simulink model "fan_control_Old"  (R2024b)
settings: Solver=VariableStepAuto  StartTime=0.0  StopTime=inf  FixedStep=1e-4  MaxStep=1e-4  RelTol=1e-6
values from neighbouring files (symbols this model uses):
  a = 0.0    [data.sldd]
  J_f = 0.0    [data.sldd]
  J_m = 0.0    [data.sldd]
  PID_I = 0.03    [data.sldd]
  PID_P = 0.06    [data.sldd]
  RateSpeed = 0.0    [data.sldd]
  RateTorque = 0.0    [data.sldd]
  Reference_Speed = 0.0    [data.sldd]
  Speed_max = 0.0    [data.sldd]
  T0 = 0.0    [data.sldd]
  Torque_max = 0.0    [data.sldd]
settings Model: DataDictionary=data.sldd  Creator=SESA504213  LastModifiedBy=SESA504213

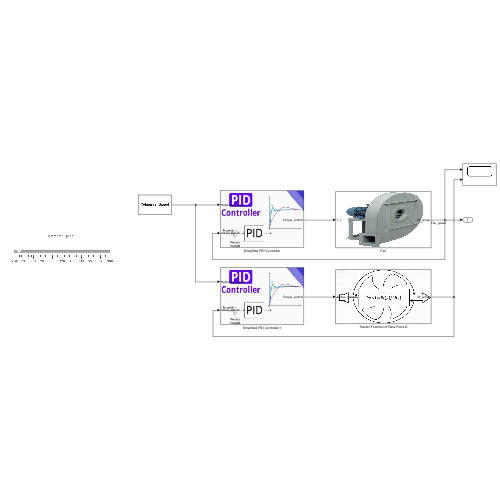
[thumbnail: Simulink's stored preview of the top-level diagram]
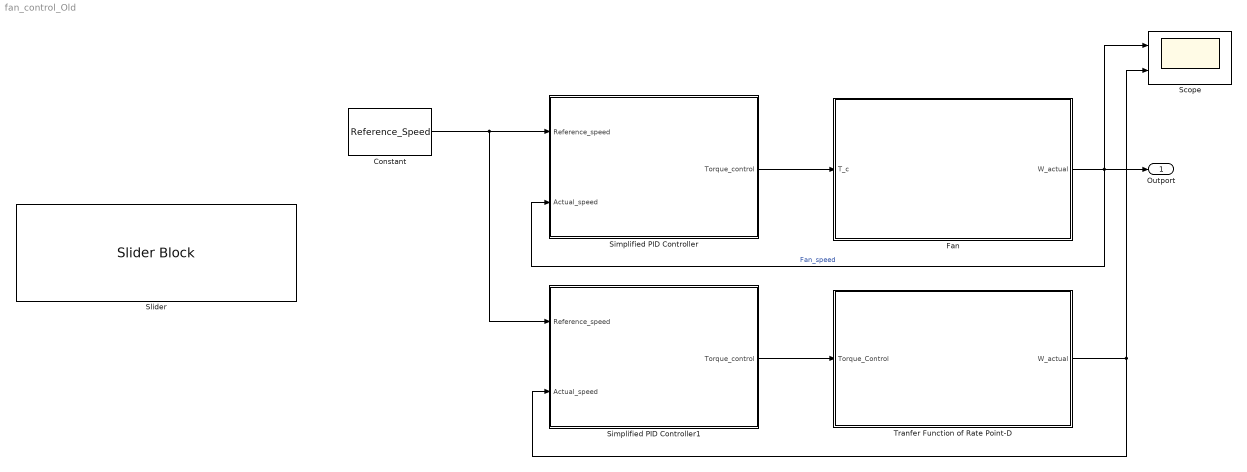
== system fan_control_Old ==
  Constant : Constant  Value=Reference_Speed
  Fan : Subsystem
      mask Display: image('FanwithMotor.jpg');
  Scope : Scope  NumInputPorts=2
  Simplified PID Controller : Subsystem
      mask Display: image('PIDController.jpg');
  Simplified PID Controller1 : Subsystem
      mask Display: image('PIDController.jpg');
  Slider : SliderBlock  ScaleMin=250  ScaleMax=390
  Tranfer Function of Rate Point-D : Subsystem
      mask Display: image('TransferFcn.jpg');
  Outport : Outport
  wires:
  Fan/1(W_actual) -> Outport/1, Simplified PID Controller/2(Actual_speed), Scope/1  "Fan_speed"
  Simplified PID Controller/1(Torque_control) -> Fan/1(T_c)
  Constant/1 -> Simplified PID Controller1/1(Reference_speed), Simplified PID Controller/1(Reference_speed)
  Simplified PID Controller1/1(Torque_control) -> Tranfer Function of Rate Point-D/1(Torque_Control)
  Tranfer Function of Rate Point-D/1(W_actual) -> Simplified PID Controller1/2(Actual_speed), Scope/2

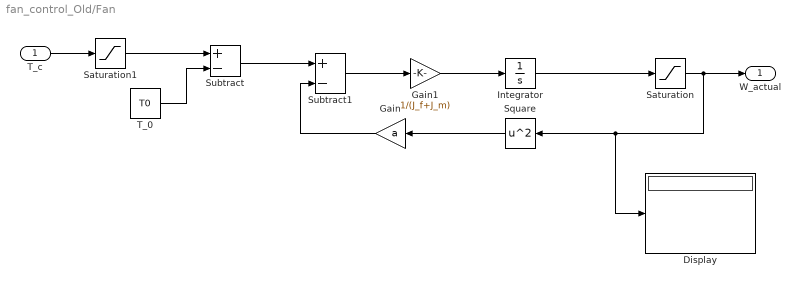
== system fan_control_Old/Fan ==
  T_c : Inport
  Display : Display
  Gain : Gain  Gain=a
  Gain1 : Gain  Gain=1/(J_f+J_m)
  Integrator : Integrator
  Saturation : Saturate  UpperLimit=Speed_max  LowerLimit=-Speed_max
  Saturation1 : Saturate  UpperLimit=Torque_max  LowerLimit=-Torque_max
  Square : Math  Operator=square
  Subtract : Sum  Inputs=+-
  Subtract1 : Sum  Inputs=+-
  T_0 : Constant  Value=T0
  W_actual : Outport
  wires:
  Gain1/1 -> Integrator/1
  Square/1 -> Gain/1
  T_c/1 -> Saturation1/1
  T_0/1 -> Subtract/2
  Subtract1/1 -> Gain1/1
  Integrator/1 -> Saturation/1
  Subtract/1 -> Subtract1/1
  Gain/1 -> Subtract1/2
  Saturation/1 -> Display/1, Square/1, W_actual/1
  Saturation1/1 -> Subtract/1

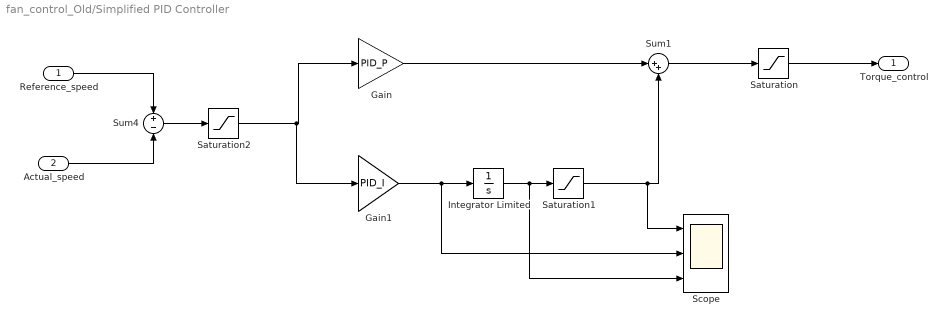
== system fan_control_Old/Simplified PID Controller ==
  Reference_speed : Inport
  Actual_speed : Inport  Port=2
  Gain : Gain  Gain=PID_P
  Gain1 : Gain  Gain=PID_I
  Integrator Limited : Integrator  LimitOutput=on  UpperSaturationLimit=RateTorque  LowerSaturationLimit=-RateTorque
  Saturation : Saturate  UpperLimit=Torque_max  LowerLimit=-Torque_max
  Saturation1 : Saturate  UpperLimit=Torque_max  LowerLimit=-Torque_max
  Saturation2 : Saturate  UpperLimit=Speed_max  LowerLimit=-Speed_max
  Scope : Scope  NumInputPorts=3
  Sum1 : Sum  Inputs=|++
  Sum4 : Sum  Inputs=+-
  Torque_control : Outport
  wires:
  Gain1/1 -> Integrator Limited/1, Scope/2
  Gain/1 -> Sum1/1
  Sum1/1 -> Saturation/1
  Integrator Limited/1 -> Scope/3, Saturation1/1
  Saturation1/1 -> Scope/1, Sum1/2
  Saturation/1 -> Torque_control/1
  Reference_speed/1 -> Sum4/1
  Actual_speed/1 -> Sum4/2
  Saturation2/1 -> Gain1/1, Gain/1
  Sum4/1 -> Saturation2/1

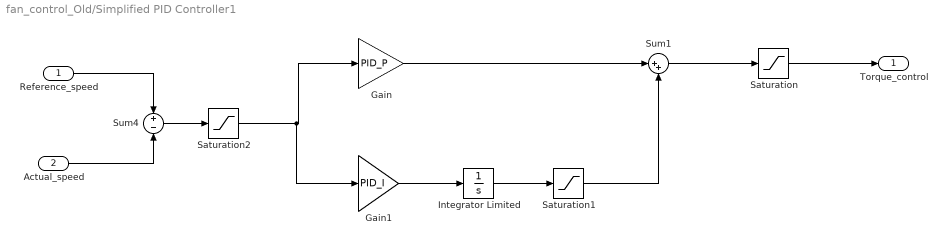
== system fan_control_Old/Simplified PID Controller1 ==
  Reference_speed : Inport
  Actual_speed : Inport  Port=2
  Gain : Gain  Gain=PID_P
  Gain1 : Gain  Gain=PID_I
  Integrator Limited : Integrator  LimitOutput=on  UpperSaturationLimit=RateTorque  LowerSaturationLimit=-RateTorque
  Saturation : Saturate  UpperLimit=Torque_max  LowerLimit=-Torque_max
  Saturation1 : Saturate  UpperLimit=Torque_max  LowerLimit=-Torque_max
  Saturation2 : Saturate  UpperLimit=Speed_max  LowerLimit=-Speed_max
  Sum1 : Sum  Inputs=|++
  Sum4 : Sum  Inputs=+-
  Torque_control : Outport
  wires:
  Gain1/1 -> Integrator Limited/1
  Gain/1 -> Sum1/1
  Sum1/1 -> Saturation/1
  Integrator Limited/1 -> Saturation1/1
  Saturation1/1 -> Sum1/2
  Saturation/1 -> Torque_control/1
  Reference_speed/1 -> Sum4/1
  Actual_speed/1 -> Sum4/2
  Saturation2/1 -> Gain1/1, Gain/1
  Sum4/1 -> Saturation2/1

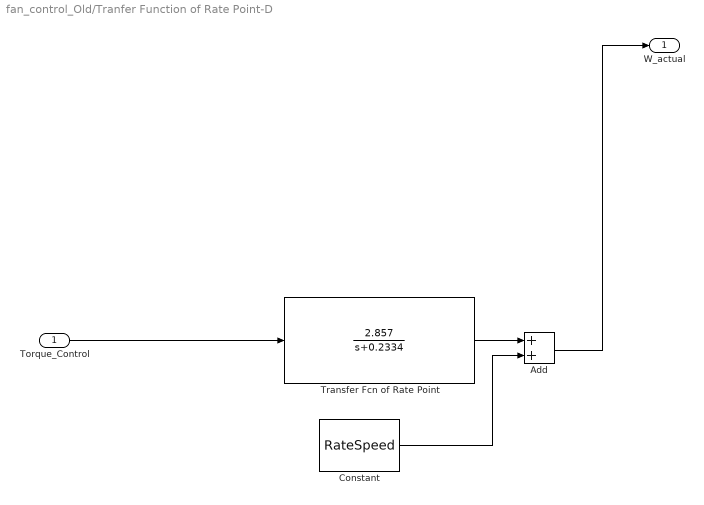
== system fan_control_Old/Tranfer Function of Rate Point-D ==
  Torque_Control : Inport
  Add : Sum
  Constant : Constant  Value=RateSpeed
  "Transfer Fcn of Rate Point " : TransferFcn  Numerator=[2.857]  Denominator=[1 0.2334]
  W_actual : Outport
  wires:
  "Transfer Fcn of Rate Point "/1 -> Add/1
  Constant/1 -> Add/2
  Torque_Control/1 -> "Transfer Fcn of Rate Point "/1
  Add/1 -> W_actual/1
